simulink model "model"  (Simulink 10.3)
settings: Solver=ode1  StartTime=0.0  StopTime=max(cyc_mph(:,1))  FixedStep=1  MaxStep=1  RelTol=1e-3  AbsTol=1e-3
undefined symbols (not defined in the file): acc_elec_eff, acc_elec_pwr, acc_mech_eff, amb_tmp, cs_charge_deplete_bool, cs_electric_decel_spd, cs_electric_launch_spd_hi, cs_electric_launch_spd_lo, cs_hi_soc, cs_lo_soc, cs_off_trq_frac, cyc_avg_time, cyc_cargo_mass, cyc_elevation_init, cyc_filter_bool, cyc_grade, cyc_mph, ess_module_num, ess_on, ess_voc, ex_calc, ex_cat_co_frac, ex_cat_ext_cp, ex_cat_ext_emisv, ex_cat_ext_init_tmp, ex_cat_ext_mass, ex_cat_ext_sarea, ex_cat_hc_frac, ex_cat_i2p_th_cond, ex_cat_i2x_emisv, ex_cat_i2x_th_cond, ex_cat_int_cp, ex_cat_int_init_tmp, ex_cat_int_mass, ex_cat_int_sarea, ex_cat_lim, ex_cat_m2i_th_cond, ex_cat_m2i_tmp, ex_cat_m2p_emisv, ex_cat_mon_cp, ex_cat_mon_init_tmp, ex_cat_mon_mass, ex_cat_mon_sarea, ex_cat_monf_sarea, ex_cat_moni_sarea, ex_cat_nox_frac, ex_cat_p2x_th_cond, ex_cat_pcm_ecp, ex_cat_pcm_mass, ex_cat_pcm_tmp, ex_cat_pipe_cp, ex_cat_pipe_emisv, ex_cat_pipe_init_tmp, ex_cat_pipe_mass, ex_cat_pipe_sarea, ex_cat_pm_frac, ex_cat_tmp_range, ex_gas_cp, ex_manif_cp, ex_manif_emisv ... (+73)
libraries: lib_controls x6, lib_vehicle x3, lib_accessory x2, lib_interactive x1, lib_energy_storage x1, lib_fuel_converter x1
(part 5 of 5)

== system model/mechanical accessory loads <acc>/Mechanical Accessory Loads v2 <acc>/backward model ==
  note: Power, W, input to accessory
  note: T, Nm, shaft out
  note: T, Nm, driveline
  note: T, Nm, accessory
  note: w_apu, rad/s
  trq_in : Inport
  spd_in : Inport  Port=2
  acc on/off : Inport  Port=3
  Product : Product  Inputs=**  InputSameDT=on  RndMeth=Zero  SaturateOnIntegerOverflow=on  OutDataTypeStr=Inherit: Same as first input
  Product1 : Product  Inputs=**  InputSameDT=on  RndMeth=Zero  SaturateOnIntegerOverflow=on  OutDataTypeStr=Inherit: Same as first input
  Sum : Sum  Inputs=|++  InputSameDT=on  SaturateOnIntegerOverflow=on  OutDataTypeStr=Inherit: Same as first input
  acc_mech_var_loads : ToWorkspace  VariableName=acc_mech_var_load  SaveFormat=Structure  SampleTime=-1
  mechanical accessories (Nm) : Subsystem  BlockChoice=Mechanical Accessories: Const Mech Var Elect
      settings: AttributesFormatString=%<BlockChoice>  TemplateBlock=lib_accessory/mechanical accessories (Nm)  MemberBlocks=Mechanical Accessories: Const Mech Var Elect,Mechanical Accessories: Constant Mechanical & Electrical,Mechanical Accessories: Speed Dependant and Variable Electrical,Saber Dual Voltage Cosim,Saber Single Voltage Cosim,SindaTransAC
      mask Display: image(imread('bdi_acc_pic_cs.bmp'))
  trq_out : Outport
  acc_mech_trq_r : Outport  Port=2
  acc_mech_pwr_r : Outport  Port=3
  wires:
  mechanical accessories (Nm)/3(probes) -> acc_mech_var_loads/1
  [acc_on] -> Product1/2
  [acc_on] -> Product/1
  acc on/off/1 -> [acc_on]
  mechanical accessories (Nm)/2(P_mech_acc) -> Product1/1
  Product1/1 -> acc_mech_pwr_r/1
  mechanical accessories (Nm)/1(T_acc) -> Product/2
  Product/1 -> Sum/2, acc_mech_trq_r/1
  Sum/1 -> trq_out/1
  trq_in/1 -> Sum/1
  spd_in/1 -> mechanical accessories (Nm)/1(w_APU)

== system model/mechanical accessory loads <acc>/Mechanical Accessory Loads v2 <acc>/forward model ==
  note: acc torque, Nm
  note: NOTES
  note: This simplistic model may not correctly account for accessory torque and/or power
      | when the upstream torque provider is torque or speed limited
  note: Power, W, input to accessory
  note: T, Nm, shaft out
  note: driveline and
      | acc torque, Nm
  note: T, Nm, accessory
  note: acc speed, rad/s
  trq_in : Inport
  spd_in : Inport  Port=2
  acc_trq_req : Inport  Port=3
  Product1 : Product  Inputs=**  InputSameDT=on  RndMeth=Zero  SaturateOnIntegerOverflow=on  OutDataTypeStr=Inherit: Same as first input
  Sum : Sum  Inputs=|+-  InputSameDT=on  SaturateOnIntegerOverflow=on  OutDataTypeStr=Inherit: Same as first input
  trq_out : Outport
  acc_mech_trq_a : Outport  Port=2
  acc_mech_pwr_a : Outport  Port=3
  wires:
  [pm_trq_a] -> Sum/1
  acc_trq_req/1 -> [acc_trq_r]
  trq_in/1 -> [pm_trq_a]
  [acc_spd] -> Product1/2
  [acc_trq_r] -> Product1/1, Sum/2, acc_mech_trq_a/1
  Product1/1 -> acc_mech_pwr_a/1
  Sum/1 -> trq_out/1
  spd_in/1 -> [acc_spd]

== system model/motor/ controller <mc> par/N-m drive torque per W input/Block NOTES ==
  note: This block determines the ratio of req'd rotor torque to req'd electrical input power,
      |  which is proportional to efficiency if the motor is providing torque.  This ratio is used
      | to compute actual rotor torque given some input power which may be different from
      | the req'd value.
      |
      | If the denominator, the req'd input power, is zero, this block outputs inf,
      | which is a flag used by the block .../rotor drive torque available (Nm).

== system model/motor/ controller <mc> par/effect of inertia (Nm)/Block NOTES ==
  note: Torque required to accelerate the motor's inertia is calculated from the rate of change
      | of mc_spd_out_a.  It is no greater than the product of the maximum motor torque and
      | the fractional contribution of the motor's inertia to the total vehicle inertia.

== system model/motor/ controller <mc> par/effect of inertia (Nm)/motor inertia as a function of total vehicle inertia (generous approximation) ==
  gear ratio : Inport
  Product : Product  Inputs=*/  SaturateOnIntegerOverflow=on
  Sum : Sum  Inputs=++|  SaturateOnIntegerOverflow=on
  engine inertia as a fraction of total vehicle inertia  (generous approximation)--denomenator : Fcn  Expr=mc_inertia*u^2
  engine inertia as a fraction of total vehicle inertia  (generous approximation)--numerator : Fcn  Expr=mc_inertia*u^2
  veh mass calc : Subsystem
  Out1 : Outport
  wires:
  Sum/1 -> Product/2
  engine inertia as a fraction of total vehicle inertia  (generous approximation)--denomenator/1 -> Sum/2
  veh mass calc/1(Out1) -> Sum/1
  gear ratio/1 -> engine inertia as a fraction of total vehicle inertia  (generous approximation)--denomenator/1, engine inertia as a fraction of total vehicle inertia  (generous approximation)--numerator/1
  Product/1 -> Out1/1
  engine inertia as a fraction of total vehicle inertia  (generous approximation)--numerator/1 -> Product/1

== system model/motor/ controller <mc> par/enforce torque limit/Block NOTES ==
  note: This block enforces the maximum torque production and absorption
      | capability limits of the motor.  It assumes that exactly as much torque
      | can be absorbed as can be produced at a given speed.

== system model/motor/ controller <mc> par/mc tmp/Block NOTES ==
  note: This block models the thermal behavior of a motor
      | and controller  with active fluid cooling.
      | The module is modeled as a single lumped thermal mass.
      | The fan is on whenever the battery temp is > the set temp.

== system model/motor/ controller <mc> par/mc tmp/mc coolant ==
  Tcl : Inport
  "Qmc " : Inport  Port=2
  Enable : EnablePort  StatesWhenEnabling=reset
  Constant : Constant  Value=mc_tstat
  Product1 : Product  SaturateOnIntegerOverflow=on
  Relational Operator : RelationalOperator  Operator=<=  RndMeth=Nearest  InputSameDT=on
  Qmc_clt : Outport  OutputWhenDisabled=reset  InitialOutput=0
  wires:
  Tcl/1 -> Relational Operator/2
  Constant/1 -> Relational Operator/1
  "Qmc "/1 -> Product1/2
  Product1/1 -> Qmc_clt/1
  Relational Operator/1 -> Product1/1

== system model/motor/ controller <mc> par/motor speed estimator/Block NOTES ==
  note: The requested motor speed is replaced by an estimate of the
      | motor's previous speed, for loss and max. torque calculations,
      | whenever the vehicle missed the trace by more than 1 mph
      | on the last time step.

== system model/motor/ controller <mc> par/rotor drive torque available (Nm)/Block NOTES ==
  note: This block computes the actual rotor torque given the actual motor input power and
      | the ratio (req'd rotor torque)/(req'd input power).
      |
      | If the above ratio has the value inf, which implies that the req'd input power is zero,
      | then the actual rotor torque is assumed to be zero.  This is not reflective of reality, of course:
      | with zero input power, the rotor torque would be the motor spin-loss torque at the given speed.
      | Because this simplification occurs only when req'd input power is zero, it does not.
      | affect fuel economy or max effort acceleration calculations.

== system model/vehicle <veh>/force req'd to accelerate (N)/current veh mass ==
  Constant3 : Constant  Value=veh_mass
  Sum1 : Sum  Inputs=|++  SaturateOnIntegerOverflow=on
  Out1 : Outport
  wires:
  Constant3/1 -> Sum1/1
  [veh_cargo_mass] -> Sum1/2
  Sum1/1 -> Out1/1

== system model/vehicle <veh>/force req'd to ascend (N)/current veh mass ==
  Constant3 : Constant  Value=veh_mass
  Sum1 : Sum  Inputs=|++  SaturateOnIntegerOverflow=on
  Out1 : Outport
  wires:
  Constant3/1 -> Sum1/1
  [veh_cargo_mass] -> Sum1/2
  Sum1/1 -> Out1/1

== system model/vehicle <veh>/record achieved force outputs/force req'd to accelerate (N)1 ==
  v(m/s) : Inport
  v prev : Inport  Port=2
  Clock : Clock
  Memory : Memory  InitialCondition=-0.1
  Product1 : Product  Inputs=**/  SaturateOnIntegerOverflow=on
  Sum : Sum  Inputs=+-  SaturateOnIntegerOverflow=on
  Sum1 : Sum  Inputs=+-  SaturateOnIntegerOverflow=on
  current veh mass : Subsystem
  (N) : Outport  InitialOutput=0
  wires:
  current veh mass/1(Out1) -> Product1/1
  Clock/1 -> Sum1/1, Memory/1
  Memory/1 -> Sum1/2
  Product1/1 -> (N)/1
  v prev/1 -> Sum/2
  v(m/s)/1 -> Sum/1
  Sum1/1 -> Product1/3
  Sum/1 -> Product1/2

== system model/vehicle <veh>/record achieved force outputs/force req'd to ascend (N)1 ==
  average vehicle speed over time step (m/s) : Inport
  Constant : Constant  Value=veh_gravity
  Constant1 : Constant  Value=0
  Product : Product  Inputs=3  SaturateOnIntegerOverflow=on
  Switch : Switch  SaturateOnIntegerOverflow=on  InputSameDT=on
  Trigonometric Function : Trigonometry  Operator=atan
  Trigonometric Function1 : Trigonometry
  current veh mass : Subsystem
  (N) : Outport  InitialOutput=0
  wires:
  current veh mass/1(Out1) -> Product/3
  average vehicle speed over time step (m/s)/1 -> Switch/2
  Constant1/1 -> Switch/3
  Switch/1 -> (N)/1
  Product/1 -> Switch/1
  Constant/1 -> Product/1
  [grade] -> Trigonometric Function/1
  Trigonometric Function1/1 -> Product/2
  Trigonometric Function/1 -> Trigonometric Function1/1

== system model/vehicle <veh>/record achieved force outputs/force req'd to overcome aerodynamic drag (N)1 ==
  average vehicle speed over time step (m/s) : Inport
  Constant : Constant  Value=veh_air_density*veh_CD*veh_FA*0.5
  Product : Product  Inputs=3  SaturateOnIntegerOverflow=on
  D aero(N) : Outport  InitialOutput=0
  wires:
  Product/1 -> D aero(N)/1
  Constant/1 -> Product/3
  average vehicle speed over time step (m/s)/1 -> Product/2, Product/1

== system model/vehicle <veh>/record achieved force outputs/rolling resistance force ==
  average vehicle speed over time step (m/s) : Inport
  force req'd to overcome rolling resistance (N) : lib_vehicle/Submodels/force req'd to overcome rolling resistance (N)  SystemSampleTime=-1  VariantActivationTime=update diagram  Latency=0  AutoFrameSizeCalculation=off
  Fr (N) : Outport
  wires:
  average vehicle speed over time step (m/s)/1 -> force req'd to overcome rolling resistance (N)/1
  force req'd to overcome rolling resistance (N)/1 -> Fr (N)/1

== system model/wheel and axle  front/rear <wh>/front force/brake request  controller interface ==
  F_front_brake_req : Outport  InitialOutput=0
  wires:
  [F_front_brake_req] -> F_front_brake_req/1

== system model/wheel and axle  front/rear <wh>/loss (Nm)/veh mass calc ==
  Constant : Constant  Value=veh_mass
  Sum : Sum  Inputs=|++  SaturateOnIntegerOverflow=on
  Out1 : Outport
  wires:
  Sum/1 -> Out1/1
  Constant/1 -> Sum/2
  [veh_cargo_mass] -> Sum/1

== system model/wheel and axle  front/rear <wh>/rear force/brake request controller interface1 ==
  F_rear_brake_req : Outport  InitialOutput=0
  wires:
  [F_rear_brake_req] -> F_rear_brake_req/1

== system model/wheel and axle  front/rear <wh>/tire slip model (m/s)/Block NOTES ==
  note: This block implements the effects of finite tire slip (with respect to the road) on the
      | vehicle speed/wheel speed relationship.  Slip is defined as s=(omega*r - v) / v.  The
      | one-to-one mapping of slip to normalized tractive force, F_tract/W_front_axle, up to
      | the maximum, is stored in the variables "wh_slip" and "wh_slip_force_coeff."  The
      | slip calculation here is overridden if the actual axle speed and the requested axle
      | speed are the same, indicating that no drivetrain speed limits were encountered.

== system model/wheel and axle  front/rear <wh>/tire slip model (m/s)/front axle ==
  In1 : Inport
  In2 : Inport  Port=2
  Abs : Abs  SaturateOnIntegerOverflow=on
  Constant3 : Constant  Value=0
  F/W : Product  Inputs=*/  SaturateOnIntegerOverflow=on
  Product : Product  SaturateOnIntegerOverflow=on
  Relational Operator : RelationalOperator  Operator=~=  RndMeth=Nearest  InputSameDT=on
  Saturation : Saturate  UpperLimit=max(wh_slip_force_coeff)  LowerLimit=min(wh_slip_force_coeff)
  Sign : Signum
  Switch : Switch  SaturateOnIntegerOverflow=on  InputSameDT=on
  s=s(F/W) : Lookup  InputValues=wh_slip_force_coeff  Table=wh_slip  SaturateOnIntegerOverflow=on
  Out1 : Outport
  wires:
  Product/1 -> Out1/1
  In1/1 -> F/W/2
  In2/1 -> Sign/1, Abs/1
  s=s(F/W)/1 -> Product/1
  Sign/1 -> Product/2
  F/W/1 -> Switch/1
  Switch/1 -> Saturation/1
  Saturation/1 -> s=s(F/W)/1
  Abs/1 -> Relational Operator/1, F/W/1
  Relational Operator/1 -> Switch/2
  Constant3/1 -> Relational Operator/2, Switch/3

== system model/wheel and axle  front/rear <wh>/tire slip model (m/s)/rear axle ==
  In1 : Inport
  In2 : Inport  Port=2
  Abs : Abs  SaturateOnIntegerOverflow=on
  Constant3 : Constant  Value=0
  F/W : Product  Inputs=*/  SaturateOnIntegerOverflow=on
  Product : Product  SaturateOnIntegerOverflow=on
  Relational Operator : RelationalOperator  Operator=~=  RndMeth=Nearest  InputSameDT=on
  Saturation : Saturate  UpperLimit=max(wh_slip_force_coeff)  LowerLimit=min(wh_slip_force_coeff)
  Sign : Signum
  Switch : Switch  SaturateOnIntegerOverflow=on  InputSameDT=on
  s=s(F/W) : Lookup  InputValues=wh_slip_force_coeff  Table=wh_slip  SaturateOnIntegerOverflow=on
  Out1 : Outport
  wires:
  Product/1 -> Out1/1
  In1/1 -> F/W/2
  In2/1 -> Sign/1, Abs/1
  s=s(F/W)/1 -> Product/1
  Sign/1 -> Product/2
  F/W/1 -> Switch/1
  Switch/1 -> Saturation/1
  Saturation/1 -> s=s(F/W)/1
  Abs/1 -> Relational Operator/1, F/W/1
  Relational Operator/1 -> Switch/2
  Constant3/1 -> Relational Operator/2, Switch/3

== system model/wheel and axle  front/rear <wh>/tire slip model (rad/s)/front slip ==
  In1 : Inport
  In2 : Inport  Port=2
  Abs : Abs  SaturateOnIntegerOverflow=on
  F/W : Product  Inputs=*/  SaturateOnIntegerOverflow=on
  Product : Product  SaturateOnIntegerOverflow=on
  Saturation : Saturate  UpperLimit=max(wh_slip_force_coeff)  LowerLimit=min(wh_slip_force_coeff)
  Sign : Signum
  s=s(F/W) : Lookup  InputValues=wh_slip_force_coeff  Table=wh_slip  SaturateOnIntegerOverflow=on
  Out1 : Outport
  wires:
  Product/1 -> Out1/1
  In1/1 -> F/W/2
  s=s(F/W)/1 -> Product/1
  In2/1 -> Sign/1, Abs/1
  Sign/1 -> Product/2
  Abs/1 -> F/W/1
  F/W/1 -> Saturation/1
  Saturation/1 -> s=s(F/W)/1

== system model/wheel and axle  front/rear <wh>/tire slip model (rad/s)/rear slip ==
  In1 : Inport
  In2 : Inport  Port=2
  Abs : Abs  SaturateOnIntegerOverflow=on
  F/W : Product  Inputs=*/  SaturateOnIntegerOverflow=on
  Product : Product  SaturateOnIntegerOverflow=on
  Saturation : Saturate  UpperLimit=max(wh_slip_force_coeff)  LowerLimit=min(wh_slip_force_coeff)
  Sign : Signum
  s=s(F/W) : Lookup  InputValues=wh_slip_force_coeff  Table=wh_slip  SaturateOnIntegerOverflow=on
  Out1 : Outport
  wires:
  Product/1 -> Out1/1
  In1/1 -> F/W/2
  s=s(F/W)/1 -> Product/1
  In2/1 -> Sign/1, Abs/1
  Sign/1 -> Product/2
  Abs/1 -> F/W/1
  F/W/1 -> Saturation/1
  Saturation/1 -> s=s(F/W)/1

== system model/<vc> par/parallel clutch control/gearbox speed estimator/Block NOTES ==
  note: The requested engine speed is replaced by an estimate of the
      | engine's previous speed whenever the vehicle missed the trace
      |  by more than 1 mph on the last time step.

== system model/<vc> par/parallel clutch control/gearbox speed estimator/dt ==
  Clock : Clock
  Memory1 : Memory  InitialCondition=-1
  Sum4 : Sum  Inputs=+-  InputSameDT=on  SaturateOnIntegerOverflow=on  OutDataTypeStr=Inherit: Same as first input
  Out1 : Outport  InitialOutput=0
  wires:
  Sum4/1 -> Out1/1
  Memory1/1 -> Sum4/2
  Clock/1 -> Memory1/1, Sum4/1

== system model/<vc> par/pre-TX parallel gearbox control/allow upshift?/Block NOTES1 ==
  note: This block prevents an upshift if it the engine is not on and
      | the upshift would make the motor power low enough that it
      | could not provide the required input power.  However, an upshift
      | is allowed if to stay in the current gear would put the motor
      | beyond 95% of its maximum speed.
      |
      | This block is to be used in pretransmission parallel hybrids
      | (where the engine and motor torques are combined on the
      | engine side of the transmission) ONLY.

== system model/<vc> par/pre-TX parallel gearbox control/downshift  command/load fraction ==
  In1 : Inport
  S-Function : S-Function  FunctionName=sfun_gearbox  Parameters=load, spd  SFunctionDeploymentMode=off  EnableBusSupport=off
  Out1 : Outport  InitialOutput=0
  wires:
  S-Function/1 -> Out1/1
  In1/1 -> S-Function/1

== system model/<vc> par/pre-TX parallel gearbox control/gearbox speed estimator/Block NOTES ==
  note: The requested engine speed is replaced by an estimate of the
      | engine's previous speed whenever the vehicle missed the trace
      |  by more than 1 mph on the last time step.

== system model/<vc> par/pre-TX parallel gearbox control/gearbox speed estimator/dt ==
  Clock : Clock
  Memory1 : Memory  InitialCondition=-1
  Sum4 : Sum  Inputs=+-  InputSameDT=on  SaturateOnIntegerOverflow=on  OutDataTypeStr=Inherit: Same as first input
  Out1 : Outport  InitialOutput=0
  wires:
  Sum4/1 -> Out1/1
  Memory1/1 -> Sum4/2
  Clock/1 -> Memory1/1, Sum4/1

== system model/<vc> par/pre-TX parallel gearbox control/shifting1/time since last shift ==
  in_1 : Inport
  just shifted : Subsystem
      mask Display: disp('just\nshifted')
  timer : Subsystem
      mask Display: disp('timer')
  out_1 : Outport  InitialOutput=0
  wires:
  timer/1(time) -> out_1/1
  just shifted/1(out_1) -> timer/1(trigger)
  in_1/1 -> just shifted/1(in_1)

== system model/<vc> par/pre-TX parallel gearbox control/upshift  command/load fraction ==
  In1 : Inport
  S-Function : S-Function  FunctionName=sfun_gearbox  Parameters=load, spd  SFunctionDeploymentMode=off  EnableBusSupport=off
  Out1 : Outport  InitialOutput=0
  wires:
  S-Function/1 -> Out1/1
  In1/1 -> S-Function/1

== system model/electric acc loads <acc>/Electrical Accessory Loads v2 <acc>/Accessory SDO/electrical power logging ==
  In1 : Inport
  Gain : Gain  Gain=acc_elec_eff  SaturateOnIntegerOverflow=on  OutDataTypeStr=Inherit: Same as input  ParamDataTypeStr=Inherit: Same as input
  To Workspace6 : ToWorkspace  VariableName=acc_elec_pwr_in_a  SampleTime=-1
  To Workspace8 : ToWorkspace  VariableName=acc_elec_pwr_out_a  SampleTime=-1
  wires:
  Gain/1 -> To Workspace8/1
  In1/1 -> Gain/1, To Workspace6/1

== system model/electric acc loads <acc>/Electrical Accessory Loads v2 <acc>/backward model/electrical accessories (W) ==
  Electrical Accessories: Time Variable : lib_accessory/Electrical Accessories: Time Variable  SystemSampleTime=-1  VariantActivationTime=update diagram  Latency=0  AutoFrameSizeCalculation=off
  P_elec_acc : Outport
  wires:
  Electrical Accessories: Time Variable/1 -> P_elec_acc/1

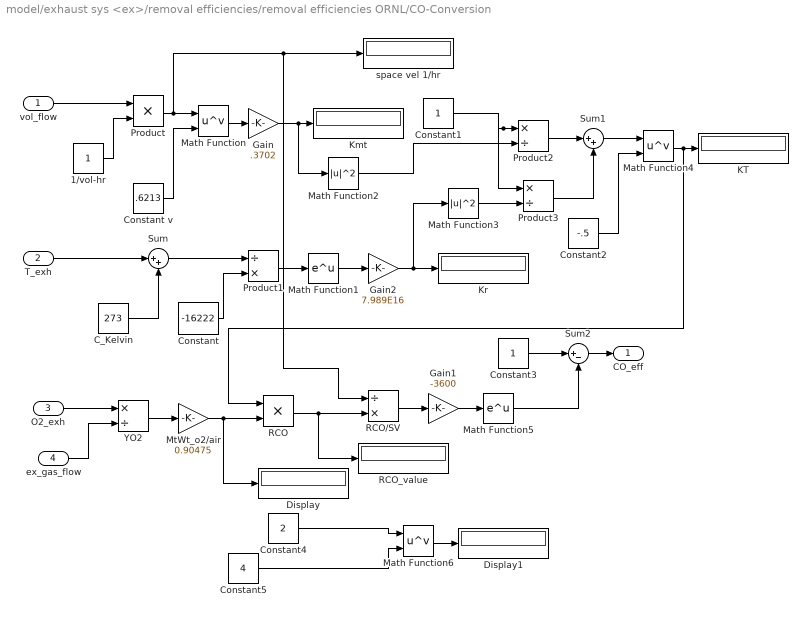
== system model/exhaust sys <ex>/removal efficiencies/removal efficiencies ORNL/CO-Conversion ==
  vol_flow : Inport
  T_exh : Inport  Port=2
  O2_exh : Inport  Port=3
  ex_gas_flow : Inport  Port=4
  1/vol-hr : Constant
  C_Kelvin : Constant  Value=273
  Constant : Constant  Value=-16222
  Constant v : Constant  Value=.6213
  Constant1 : Constant
  Constant2 : Constant  Value=-.5
  Constant3 : Constant
  Constant4 : Constant  Value=2
  Constant5 : Constant  Value=4
  Display : Display
  Display1 : Display
  Gain : Gain  Gain=.3702  SaturateOnIntegerOverflow=on
  Gain1 : Gain  Gain=-3600  SaturateOnIntegerOverflow=on
  Gain2 : Gain  Gain=7.989E16  SaturateOnIntegerOverflow=on
  KT : Display
      settings: Format=short_e
  Kmt : Display
      settings: Format=short_e
  Kr : Display
  Math Function : Math  Operator=pow  SaturateOnIntegerOverflow=on
  Math Function1 : Math  SaturateOnIntegerOverflow=on
  Math Function2 : Math  Operator=magnitude^2  SaturateOnIntegerOverflow=on
  Math Function3 : Math  Operator=magnitude^2  SaturateOnIntegerOverflow=on
  Math Function4 : Math  Operator=pow  SaturateOnIntegerOverflow=on
  Math Function5 : Math  SaturateOnIntegerOverflow=on
  Math Function6 : Math  Operator=pow  SaturateOnIntegerOverflow=on
  MtWt_o2/air : Gain  Gain=0.90475  SaturateOnIntegerOverflow=on
  Product : Product  SaturateOnIntegerOverflow=on
  Product1 : Product  Inputs=/*  SaturateOnIntegerOverflow=on
  Product2 : Product  Inputs=*/  SaturateOnIntegerOverflow=on
  Product3 : Product  Inputs=*/  SaturateOnIntegerOverflow=on
  RCO : Product  SaturateOnIntegerOverflow=on
  RCO/SV : Product  Inputs=/*  SaturateOnIntegerOverflow=on
  RCO_value : Display
  Sum : Sum  Inputs=|++  SaturateOnIntegerOverflow=on
  Sum1 : Sum  Inputs=|++  SaturateOnIntegerOverflow=on
  Sum2 : Sum  Inputs=|+-  SaturateOnIntegerOverflow=on
  YO2 : Product  Inputs=*/  SaturateOnIntegerOverflow=on
  space vel 1/hr : Display
      settings: Format=short_e
  CO_eff : Outport
  wires:
  Math Function6/1 -> Display1/1
  Constant5/1 -> Math Function6/2
  Constant4/1 -> Math Function6/1
  MtWt_o2/air/1 -> Display/1, RCO/2
  YO2/1 -> MtWt_o2/air/1
  RCO/1 -> RCO_value/1, RCO/SV/2
  Sum2/1 -> CO_eff/1
  Math Function5/1 -> Sum2/2
  Constant3/1 -> Sum2/1
  Gain1/1 -> Math Function5/1
  RCO/SV/1 -> Gain1/1
  Math Function4/1 -> RCO/1, KT/1
  ex_gas_flow/1 -> YO2/2
  O2_exh/1 -> YO2/1
  T_exh/1 -> Sum/1
  vol_flow/1 -> Product/1
  Product1/1 -> Math Function1/1
  Constant2/1 -> Math Function4/2
  Sum1/1 -> Math Function4/1
  Product3/1 -> Sum1/2
  Product2/1 -> Sum1/1
  Math Function3/1 -> Product3/2
  Math Function2/1 -> Product2/2
  Constant1/1 -> Product2/1, Product3/1
  Gain2/1 -> Math Function3/1, Kr/1
  Gain/1 -> Math Function2/1, Kmt/1
  Math Function1/1 -> Gain2/1
  Sum/1 -> Product1/1
  Constant/1 -> Product1/2
  C_Kelvin/1 -> Sum/2
  Product/1 -> RCO/SV/1, space vel 1/hr/1, Math Function/1
  Math Function/1 -> Gain/1
  Constant v/1 -> Math Function/2
  1/vol-hr/1 -> Product/2

== system model/exhaust sys <ex>/removal efficiencies/removal efficiencies ORNL/HC-Conversion ==
  vol_flow : Inport
  T_exh : Inport  Port=2
  O2_exh : Inport  Port=3
  ex_gas_flow : Inport  Port=4
  1/vol-hr : Constant
  C_Kelvin : Constant  Value=273
  Constant : Constant  Value=-10956
  Constant v : Constant  Value=.6436
  Constant2 : Constant  Value=-.1
  Constant3 : Constant
  Constant4 : Constant  Value=-2171
  Constant5 : Constant  Value=5.818
  Constant6 : Constant  Value=-10
  Gain1 : Gain  Gain=-3600  SaturateOnIntegerOverflow=on
  Gain2 : Gain  Gain=3.731E11  SaturateOnIntegerOverflow=on
  KT : Display
      settings: Format=short_e
  Kmt : Display
      settings: Format=short_e
  Kr : Display
  Math Function{,2..4} (4 alike) : Math  Operator=pow  SaturateOnIntegerOverflow=on
  Math Function1 : Math  SaturateOnIntegerOverflow=on
  Math Function5 : Math  SaturateOnIntegerOverflow=on
  Math Function6 : Math  SaturateOnIntegerOverflow=on
  MtWt_o2/air : Gain  Gain=0.90475  SaturateOnIntegerOverflow=on
  Product : Product  SaturateOnIntegerOverflow=on
  Product1 : Product  Inputs=/*  SaturateOnIntegerOverflow=on
  Product4 : Product  Inputs=*/  SaturateOnIntegerOverflow=on
  Product5 : Product  Inputs=3  SaturateOnIntegerOverflow=on
  RHC : Product  SaturateOnIntegerOverflow=on
  RHC/SV : Product  Inputs=/*  SaturateOnIntegerOverflow=on
  RHC_value : Display
  Sum : Sum  Inputs=|++  SaturateOnIntegerOverflow=on
  Sum1 : Sum  Inputs=|++  SaturateOnIntegerOverflow=on
  Sum2 : Sum  Inputs=|+-  SaturateOnIntegerOverflow=on
  YO2 : Product  Inputs=*/  SaturateOnIntegerOverflow=on
  space vel 1/hr : Display
      settings: Format=short_e
  HC_eff : Outport
  wires:
  Sum/1 -> Product4/2, Product1/1
  T_exh/1 -> Sum/1
  Math Function3/1 -> Sum1/2
  Math Function2/1 -> Sum1/1
  Constant6/1 -> Math Function3/2, Math Function2/2
  Math Function6/1 -> Product5/3
  Constant5/1 -> Product5/1
  Product4/1 -> Math Function6/1
  Constant4/1 -> Product4/1
  RHC/1 -> RHC_value/1, RHC/SV/2
  MtWt_o2/air/1 -> RHC/2
  YO2/1 -> MtWt_o2/air/1
  Sum2/1 -> HC_eff/1
  Math Function5/1 -> Sum2/2
  Constant3/1 -> Sum2/1
  Gain1/1 -> Math Function5/1
  RHC/SV/1 -> Gain1/1
  Math Function4/1 -> RHC/1, KT/1
  ex_gas_flow/1 -> YO2/2
  O2_exh/1 -> YO2/1
  vol_flow/1 -> Product/1
  Product1/1 -> Math Function1/1
  Constant2/1 -> Math Function4/2
  Sum1/1 -> Math Function4/1
  Gain2/1 -> Math Function3/1, Kr/1
  Product5/1 -> Math Function2/1, Kmt/1
  Math Function1/1 -> Gain2/1
  Constant/1 -> Product1/2
  C_Kelvin/1 -> Sum/2
  Product/1 -> RHC/SV/1, space vel 1/hr/1, Math Function/1
  Math Function/1 -> Product5/2
  Constant v/1 -> Math Function/2
  1/vol-hr/1 -> Product/2

== system model/exhaust sys <ex>/removal efficiencies/removal efficiencies ORNL/NOx_Eff ==
  vol_flow : Inport
  Ex_temp : Inport  Port=2
  HC_Inlet : Inport  Port=3
  NOx_Inlet : Inport  Port=4
  1 : Constant
  >eps : Saturate  UpperLimit=inf  LowerLimit=eps
  Gain : Gain  Gain=2.875  SaturateOnIntegerOverflow=on
  Gain1 : Gain  Gain=.01  SaturateOnIntegerOverflow=on
  HNR : Product  Inputs=*/  SaturateOnIntegerOverflow=on
  HNR^.5 : Math  Operator=sqrt  SaturateOnIntegerOverflow=on
  HNR^2 : Math  Operator=square  SaturateOnIntegerOverflow=on
  HNR^3 : Product  SaturateOnIntegerOverflow=on
  NOx_conv2 : Display
  SV^.5 : Math  Operator=sqrt  SaturateOnIntegerOverflow=on
  SV^2 : Math  Operator=square  SaturateOnIntegerOverflow=on
  SV^3 : Product  SaturateOnIntegerOverflow=on
  Saturation : Saturate  UpperLimit=1.0  LowerLimit=0.0
  Sum : Sum  Inputs=|+++++  SaturateOnIntegerOverflow=on
  Sum1 : Sum  Inputs=|++++  SaturateOnIntegerOverflow=on
  Sum2 : Sum  Inputs=|++++  SaturateOnIntegerOverflow=on
  Sum3 : Sum  Inputs=|+++  SaturateOnIntegerOverflow=on
  TR : Product  Inputs=*/  SaturateOnIntegerOverflow=on
  T^-.5 : Math  Operator=sqrt  SaturateOnIntegerOverflow=on
  T^-2 : Math  Operator=square  SaturateOnIntegerOverflow=on
  T^-3 : Product  SaturateOnIntegerOverflow=on
  b0 : Constant  Value=-1.2477959e2
  b1 : Gain  Gain=-6.671239E-4  SaturateOnIntegerOverflow=on
  b10 : Gain  Gain=-1.7874225E1  SaturateOnIntegerOverflow=on
  b11 : Gain  Gain=-2.0607707  SaturateOnIntegerOverflow=on
  b12 : Gain  Gain=1.3883777E-1  SaturateOnIntegerOverflow=on
  b13 : Gain  SaturateOnIntegerOverflow=on
  b2 : Gain  Gain=8.308073E-2  SaturateOnIntegerOverflow=on
  b3 : Gain  Gain=7.9852675E-9  SaturateOnIntegerOverflow=on
  b4 : Gain  Gain=-3.7023358E-14  SaturateOnIntegerOverflow=on
  b5 : Gain  Gain=-5.4929168E4  SaturateOnIntegerOverflow=on
  b6 : Gain  Gain=4.9229015e3  SaturateOnIntegerOverflow=on
  b7 : Gain  Gain=2.959987e6  SaturateOnIntegerOverflow=on
  b8 : Gain  Gain=-1.022441e8  SaturateOnIntegerOverflow=on
  b9 : Gain  Gain=1.3710201E1  SaturateOnIntegerOverflow=on
  NOx_eff : Outport
  wires:
  >eps/1 -> HNR/2
  NOx_Inlet/1 -> >eps/1
  Saturation/1 -> NOx_eff/1, NOx_conv2/1
  Ex_temp/1 -> TR/2
  HC_Inlet/1 -> HNR/1
  b13/1 -> SV^3/1, b1/1, SV^2/1, SV^.5/1
  Gain1/1 -> Saturation/1
  Sum3/1 -> Gain1/1
  Gain/1 -> HNR^2/1, HNR^3/2, b9/1, HNR^.5/1
  HNR/1 -> Gain/1
  Sum/1 -> Sum3/1
  Sum1/1 -> Sum3/2
  Sum2/1 -> Sum3/3
  b12/1 -> Sum2/4
  b11/1 -> Sum2/3
  b10/1 -> Sum2/2
  b9/1 -> Sum2/1
  HNR^.5/1 -> b10/1
  HNR^2/1 -> b11/1, HNR^3/1
  HNR^3/1 -> b12/1
  b8/1 -> Sum1/4
  b7/1 -> Sum1/3
  b6/1 -> Sum1/2
  b5/1 -> Sum1/1
  T^-.5/1 -> b6/1
  T^-2/1 -> b7/1, T^-3/1
  T^-3/1 -> b8/1
  TR/1 -> b5/1, T^-3/2, T^-2/1, T^-.5/1
  1/1 -> TR/1
  b3/1 -> Sum/5
  b4/1 -> Sum/4
  b1/1 -> Sum/3
  b2/1 -> Sum/2
  b0/1 -> Sum/1
  SV^.5/1 -> b2/1
  SV^2/1 -> b3/1, SV^3/2
  SV^3/1 -> b4/1
  vol_flow/1 -> b13/1

== system model/fuel converter  <fc>/engine speed estimator/no-lag Reset Integrator/dt ==
  Clock : Clock
  Memory1 : Memory  InitialCondition=-0.1
  Sum1 : Sum  Inputs=+-  InputSameDT=on  SaturateOnIntegerOverflow=on  OutDataTypeStr=Inherit: Same as first input
  out_1 : Outport  InitialOutput=0
  wires:
  Sum1/1 -> out_1/1
  Memory1/1 -> Sum1/2
  Clock/1 -> Memory1/1, Sum1/1

== system model/fuel converter  <fc>/engine torque/effect of inertia (Nm)/Block NOTES ==
  note: Torque required to accelerate the engine inertia is taken from the engine
      | acceleration, and is assumed to be no less than zero if the trace was missed
      | at all on the previous time step.
      |
      | The torque required to accelerate the engine's inertia is never assumed to
      | be more than the product of the engine's maximum torque and the engine's
      | contribution to the total vehicle inertia.

== system model/fuel converter  <fc>/engine torque/effect of inertia (Nm)/engine inertia as a function of total vehicle inertia (generous approximation) ==
  Product : Product  Inputs=*/  InputSameDT=on  RndMeth=Zero  SaturateOnIntegerOverflow=on  OutDataTypeStr=Inherit: Same as first input
  Sum : Sum  Inputs=++|  InputSameDT=on  SaturateOnIntegerOverflow=on  OutDataTypeStr=Inherit: Same as first input
  engine inertia as a fraction of total vehicle inertia  (generous approximation)--denomenator : Fcn  Expr=fc_inertia*(u*fd_ratio/wh_radius)^2
  engine inertia as a fraction of total vehicle inertia  (generous approximation)--numerator : Fcn  Expr=fc_inertia*(u*fd_ratio/wh_radius)^2
  veh mass calc : Subsystem
  Out1 : Outport
  wires:
  [gear_ratio] -> engine inertia as a fraction of total vehicle inertia  (generous approximation)--numerator/1, engine inertia as a fraction of total vehicle inertia  (generous approximation)--denomenator/1
  veh mass calc/1(Out1) -> Sum/1
  engine inertia as a fraction of total vehicle inertia  (generous approximation)--denomenator/1 -> Sum/2
  engine inertia as a fraction of total vehicle inertia  (generous approximation)--numerator/1 -> Product/1
  Sum/1 -> Product/2
  Product/1 -> Out1/1

== system model/gearbox <gb>/Pout/Pin, neglecting inertia/make division bombproof/Block NOTES ==
  note: this block added 10 July 2001 by mpo:
      | originally a -eps was added to the denominator by default.
      | However, cases were ecountered where Tin-Tineratia was equal to -eps causing
      | the denominator to be zero. This added checking is more rhobust

== system model/mechanical accessory loads <acc>/Mechanical Accessory Loads v2 <acc>/Accessory SDO/mechanical power logging ==
  In1 : Inport
  Gain : Gain  Gain=acc_mech_eff  SaturateOnIntegerOverflow=on  OutDataTypeStr=Inherit: Same as input  ParamDataTypeStr=Inherit: Same as input
  To Workspace6 : ToWorkspace  VariableName=acc_mech_pwr_in_a  SampleTime=-1
  To Workspace8 : ToWorkspace  VariableName=acc_mech_pwr_out_a  SampleTime=-1
  wires:
  Gain/1 -> To Workspace8/1
  In1/1 -> Gain/1, To Workspace6/1

== system model/mechanical accessory loads <acc>/Mechanical Accessory Loads v2 <acc>/backward model/mechanical accessories (Nm) ==
  w_APU : Inport
  Mechanical Accessories: Const Mech Var Elect : lib_accessory/Mechanical Accessories: Const Mech Var Elect  SystemSampleTime=-1  VariantActivationTime=update diagram  Latency=0  AutoFrameSizeCalculation=off
  T_acc : Outport
  P_mech_acc : Outport  Port=2
  probes : Outport  Port=3
  wires:
  w_APU/1 -> Mechanical Accessories: Const Mech Var Elect/1
  Mechanical Accessories: Const Mech Var Elect/1 -> T_acc/1
  Mechanical Accessories: Const Mech Var Elect/2 -> P_mech_acc/1
  Mechanical Accessories: Const Mech Var Elect/3 -> probes/1

== system model/motor/ controller <mc> par/effect of inertia (Nm)/motor inertia as a function of total vehicle inertia (generous approximation)/veh mass calc ==
  Constant : Constant  Value=veh_mass
  Sum : Sum  Inputs=|++  SaturateOnIntegerOverflow=on
  Out1 : Outport
  wires:
  Sum/1 -> Out1/1
  Constant/1 -> Sum/2
  [veh_cargo_mass] -> Sum/1

== system model/vehicle <veh>/record achieved force outputs/force req'd to accelerate (N)1/current veh mass ==
  Constant3 : Constant  Value=veh_mass
  Sum1 : Sum  Inputs=|++  SaturateOnIntegerOverflow=on
  Out1 : Outport
  wires:
  Constant3/1 -> Sum1/1
  [veh_cargo_mass] -> Sum1/2
  Sum1/1 -> Out1/1

== system model/vehicle <veh>/record achieved force outputs/force req'd to ascend (N)1/current veh mass ==
  Constant3 : Constant  Value=veh_mass
  Sum1 : Sum  Inputs=|++  SaturateOnIntegerOverflow=on
  Out1 : Outport
  wires:
  Constant3/1 -> Sum1/1
  [veh_cargo_mass] -> Sum1/2
  Sum1/1 -> Out1/1

== system model/<vc> par/pre-TX parallel gearbox control/shifting1/time since last shift/just shifted ==
  in_1 : Inport
  Memory : Memory  InitialCondition=1
  Relational Operator : RelationalOperator  Operator=~=  RndMeth=Nearest  InputSameDT=on
  out_1 : Outport  InitialOutput=0
  wires:
  in_1/1 -> Memory/1, Relational Operator/2
  Memory/1 -> Relational Operator/1
  Relational Operator/1 -> out_1/1

== system model/<vc> par/pre-TX parallel gearbox control/shifting1/time since last shift/timer ==
  trigger : Inport
  Constant : Constant
  Constant1 : Constant  Value=0
  Constant2 : Constant  Value=0
  Switch : Switch  Threshold=eps  SaturateOnIntegerOverflow=on  InputSameDT=on
  no-lag Reset Integrator : Subsystem  mask(No-lag Reset Integrator){initval=15}
      mask prompts: initval "Initial Value"
      mask help: No-lag Reset Integrator
      mask Help: Integrates first input using Euler technique.\nAt the time step that input 2 <> zero,\noutput is reset to input 3.
      mask Display: disp('1/s\nw/ reset\nno lag')
  time : Outport  InitialOutput=0
  wires:
  no-lag Reset Integrator/1(out_1) -> Switch/3
  Constant1/1 -> no-lag Reset Integrator/3(in_3)
  Constant/1 -> no-lag Reset Integrator/1(in_1)
  Constant2/1 -> Switch/1
  trigger/1 -> no-lag Reset Integrator/2(in_2), Switch/2
  Switch/1 -> time/1

== system model/fuel converter  <fc>/engine torque/effect of inertia (Nm)/engine inertia as a function of total vehicle inertia (generous approximation)/veh mass calc ==
  Constant : Constant  Value=veh_mass
  Sum : Sum  Inputs=|++  InputSameDT=on  SaturateOnIntegerOverflow=on  OutDataTypeStr=Inherit: Same as first input
  Out1 : Outport
  wires:
  Sum/1 -> Out1/1
  Constant/1 -> Sum/2
  [veh_cargo_mass] -> Sum/1

== system model/<vc> par/pre-TX parallel gearbox control/shifting1/time since last shift/timer/no-lag Reset Integrator ==
  in_1 : Inport
  in_2 : Inport  Port=2
  in_3 : Inport  Port=3
  Constant : Constant  Value=0
  Memory : Memory  InitialCondition=initval
  Product : Product  InputSameDT=on  RndMeth=Zero  SaturateOnIntegerOverflow=on  OutDataTypeStr=Inherit: Same as first input
  Sum : Sum  InputSameDT=on  SaturateOnIntegerOverflow=on  OutDataTypeStr=Inherit: Same as first input
  Switch : Switch  Threshold=eps  SaturateOnIntegerOverflow=on  InputSameDT=on
  dt : Subsystem
  in_2==0 : RelationalOperator  Operator===  RndMeth=Nearest  InputSameDT=on
  out_1 : Outport  InitialOutput=0
  wires:
  Constant/1 -> in_2==0/2
  in_2==0/1 -> Switch/2
  Switch/1 -> Memory/1, out_1/1
  Sum/1 -> Switch/1
  Memory/1 -> Sum/1
  Product/1 -> Sum/2
  dt/1(out_1) -> Product/1
  in_1/1 -> Product/2
  in_2/1 -> in_2==0/1
  in_3/1 -> Switch/3

== system model/<vc> par/pre-TX parallel gearbox control/shifting1/time since last shift/timer/no-lag Reset Integrator/dt ==
  Clock : Clock
  Memory1 : Memory  InitialCondition=-1
  Sum1 : Sum  Inputs=+-  InputSameDT=on  SaturateOnIntegerOverflow=on  OutDataTypeStr=Inherit: Same as first input
  out_1 : Outport  InitialOutput=0
  wires:
  Sum1/1 -> out_1/1
  Memory1/1 -> Sum1/2
  Clock/1 -> Memory1/1, Sum1/1
